simulink model "SPM_CellHarness"  (R2024b)
settings: Solver=ode15s  StartTime=0.0  StopTime=3600  FixedStep=1  MaxStep=1  RelTol=1e-4  AbsTol=1e-6
libraries: fl_lib x9, nesl_utility x5, BatteryCurrentManagement x1, batt_lib x1, BatteryEstimators x1
settings Model: Creator=annaf  LastModifiedBy=annaf

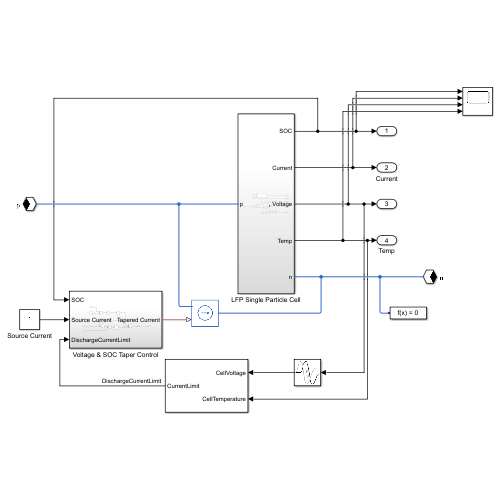
[thumbnail: Simulink's stored preview of the top-level diagram]
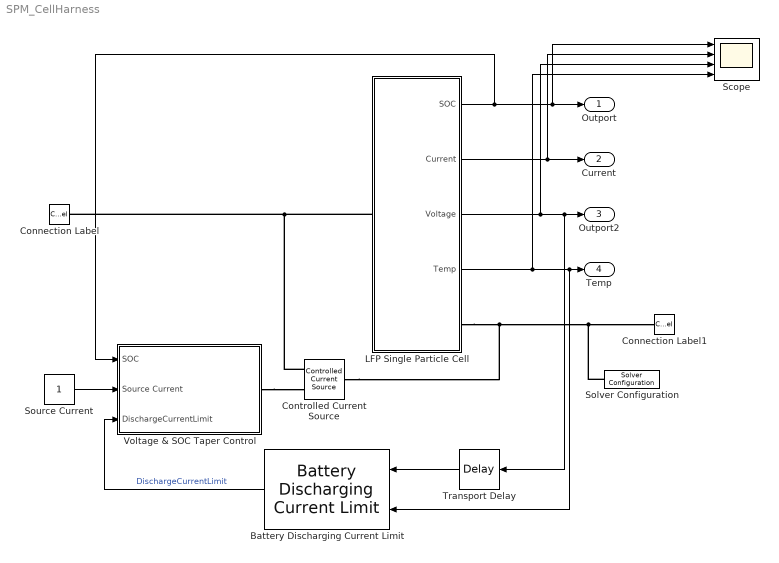
== system SPM_CellHarness ==
  Battery Discharging Current Limit : BatteryCurrentManagement/Battery Discharging Current Limit  CellUndervoltageLimit=3.2  R0=0.004  T_vec=[243.15, 258.15, 273.15, 288.15, 303.15, 318.15, 333.15]  CurrentLimitCoolestCell=[ 0, 0, 0, 0, 5, 5, 5]  CurrentLimitHottestCell=[5, 5, 5, 5, 0, 0, 0]
      settings: LibrarySourceBlock=|
      | batt_sl_lib/Current Management/Battery Discharging
      | Current Limit
  Connection Label : ConnectionLabel  Label=p
  Connection Label1 : ConnectionLabel  Label=n
  Controlled Current Source : fl_lib/Electrical/Electrical Sources/Controlled Current Source
  LFP Single Particle Cell : Subsystem
  Scope : Scope  NumInputPorts=4
  Solver Configuration : nesl_utility/Solver Configuration  PhysicalDomain=network_engine_domain  SubClassName=solver  LeftPortType=input  RightPortType=generic  Tones=[]  Harmonics=[]  SimulateNoise=off  Profile=off  UseLocalSampling=off  EnableSwitchedLinearOptims=on  FrequencyDomain=off  UseCCode=off  RelTol=0.001  AbsTol=0.001  MinStep=1e-09  ToWorkspace=off  RevertToSquareIcSolve=off  NumHomotopyIterations=100  PhasorMode=off  PhasorModeNumHarmonics=1  ConsistencySolver=NEWTON_XTOL_AFTER_FTOL  IndexReductionMethod=DerivativeReplacement  DoDC=off  ResidualTolerance=1e-09  ConsistencyTolSource=LOCAL  ConsistencyAbsTol=0.000001  ConsistencyRelTol=0.0001  ConsistencyTolFactor=0.001  UseLocalSolver=off  LocalSolverChoice=NE_BACKWARD_EULER_ADVANCER  ResolveIndetEquations=on  FunctionEvalNumThread=1  LocalSolverSampleTime=1  DoFixedCost=on  MaxNonlinIter=6  MaxModeIter=2  ComputeImpulses=off  ImpulseIterations=2  LinearAlgebra=Full  LinearAlgebraNumThread=0  EquationFormulation=NE_TIME_EF  DelaysMemoryBudget=1024  AutomaticFiltering=on  FilteringTimeConstant=0.001  PartitionStorageMethod=AS_NEEDED  PartitionMemoryBudget=1024  PartitionMethod=ROBUST  MultibodyUseLocalSolver=off  MultibodyLocalSolverChoice=ODE1  MultibodyLocalSolverSampleTime=0.001
  Source Current : Constant
  Transport Delay : TransportDelay  DelayTime=1e-6  TransDelayFeedthrough=on
  Voltage & SOC Taper Control : Subsystem
  Outport : Outport
  Current : Outport  Port=2
  Outport2 : Outport  Port=3
  Temp : Outport  Port=4
  wires:
  LFP Single Particle Cell/3(Voltage) -> Scope/3, Transport Delay/1, Outport2/1
  LFP Single Particle Cell/1(SOC) -> Scope/1, Outport/1, Voltage & SOC Taper Control/1(SOC)
  LFP Single Particle Cell/2(Current) -> Scope/2, Current/1
  LFP Single Particle Cell/4(Temp) -> Battery Discharging Current Limit/2, Temp/1, Scope/4
  Transport Delay/1 -> Battery Discharging Current Limit/1
  Battery Discharging Current Limit/1 -> Voltage & SOC Taper Control/3(DischargeCurrentLimit)  "DischargeCurrentLimit"
  Source Current/1 -> Voltage & SOC Taper Control/2(Source Current)
  connections:
  LFP Single Particle Cell/RConn1 -- Controlled Current Source/LConn1 -- Solver Configuration/RConn1 -- Connection Label1/LConn1
  LFP Single Particle Cell/LConn1 -- Controlled Current Source/RConn2 -- Connection Label/LConn1
  Voltage & SOC Taper Control/RConn1 -- Controlled Current Source/RConn1

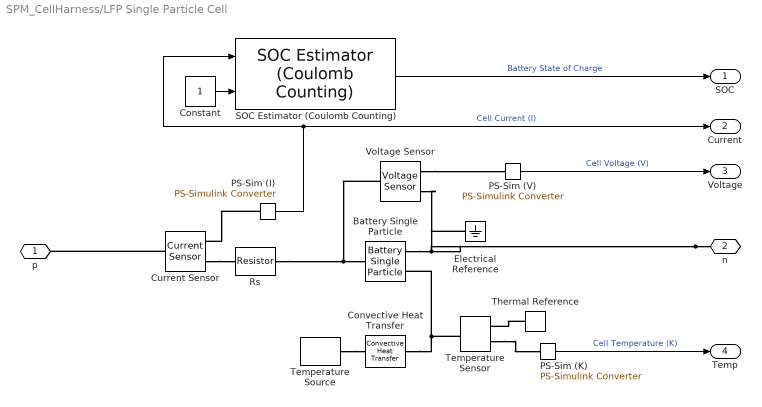
== system SPM_CellHarness/LFP Single Particle Cell ==
  Battery Single Particle : batt_lib/Cells/Electrochemical/Battery Single Particle  ExtrapolationMethod=simscape.enum.extrapolation.nearest  ThicknessAnode=3.4E-5 m  ElectrolyteLayerCountAnode=10  ThicknessSeparator=2.5E-5 m  ElectrolyteLayerCountSeparator=5  ThicknessCathode=8E-5 m  ElectrolyteLayerCountCathode=10  ElectrodePlateArea=1.5 m^2  ParticleRadiusAnode=5E-6 m  ShellCountAnode=40  ParticleRadiusCathode=5E-6 m  ShellCountCathode=40  ActiveMaterialVolumeFractionAnode=0.58  ActiveMaterialVolumeFractionCathode=0.374  OpenCircuitPotentialAnode=[0.200;0.180;0.160;0.140;0.120;0.110;0.102;0.098;0.094;0.092;0.091;0.090;0.089;0.089;0.088;0.088;0.088;0.088;0.088;0.088;0.088;0.087;0.087;0.087;0.086;0.086;0.085;0.085;0.084;0.084;0.083;0.083;0.082;0.082;0.081;0.081;0.080;0.079;0.078] V  OpenCircuitPotentialCathode=[3.200;3.280;3.340;3.380;3.410;3.420;3.425;3.430;3.432;3.433;3.434;3.435;3.435;3.436;3.436;3.437;3.437;3.438;3.438;3.439;3.439;3.440;3.440;3.441;3.441;3.442;3.442;3.443;3.443;3.444;3.444;3.445;3.446;3.447;3.448;3.449;3.460;3.480;3.500] V  NormalizedStoichiometryBreakpoints=linspace(0.025, 0.975, 39)  MaximumConcentrationAnode=30555 mol/m^3  MaximumStoichiometryAnode=0.811  MinimumStoichiometryAnode=0.0132  MaximumConcentrationCathode=22806 mol/m^3  MaximumStoichiometryCathode=0.74  MinimumStoichiometryCathode=0.035  ActiveMaterialDiffusionCoefficientAnode=3E-15 m^2/s  ActiveMaterialDiffusionCoefficientCathode=1E-15 m^2/s  ConductivityAnode=100 S/m  ConductivityCathode=0.5 S/m  CurrentCollectorResistance=1E-3 Ohm  ElectrolyteVolumeFractionAnode=0.3874  ElectrolyteVolumeFractionSeparator=0.45  ElectrolyteVolumeFractionCathode=0.5725  ElectrolyteConductivity=0.29 S/m  BruggemanExponentAnode=1.5  BruggemanExponentSeparator=1.5  BruggemanExponentCathode=1.5  TransferenceNumber=0.363  ElectrolyteDiffusionCoefficient=2E-10 m^2/s  ChargeTransferRateAnode=1E-9 m^(5/2)/(mol^(1/2)*s)  ChargeTransferRateCathode=1E-11 m^(5/2)/(mol^(1/2)*s)  BatteryThermalMass=77 J/K  ArrheniusReferenceTemperature=298.15 K  ActiveMaterialDiffusionActivationEnergyAnode=39000 J/mol  ActiveMaterialDiffusionActivationEnergyCathode=35000 J/mol  ElectrolyteDiffusionActivationEnergy=26600 J/mol  ConductivityActivationEnergyAnode=3000 J/mol  ConductivityActivationEnergyCathode=3000 J/mol  ElectrolyteConductivityActivationEnergy=11000 J/mol  ChargeTransferActivationEnergyAnode=13000 J/mol  ChargeTransferActivationEnergyCathode=20000 J/mol  batteryCurrent_specify=off  batteryCurrent_priority=None  batteryCurrent=0 A  batteryCurrent_nominal_specify=off  batteryCurrent_nominal_value=1  batteryCurrent_nominal_unit=A  batteryVoltage_specify=off  batteryVoltage_priority=None  batteryVoltage=0 V  batteryVoltage_nominal_specify=off  batteryVoltage_nominal_value=1  batteryVoltage_nominal_unit=V  averageElectrolyteConcentration_specify=off  averageElectrolyteConcentration_priority=High  averageElectrolyteConcentration=1200 mol/m^3  averageElectrolyteConcentration_nominal_specify=off  averageElectrolyteConcentration_nominal_value=1  averageElectrolyteConcentration_nominal_unit=mol/m^3  stateOfCharge_specify=off  stateOfCharge_priority=High  stateOfCharge=0.5  stateOfCharge_nominal_specify=off  stateOfCharge_nominal_value=1  stateOfCharge_nominal_unit=1  batteryTemperature_specify=off  batteryTemperature_priority=High  batteryTemperature=298.15 K  batteryTemperature_nominal_specify=off  batteryTemperature_nominal_value=1  batteryTemperature_nominal_unit=K
      settings: InternalSimscapePortConfiguration="{\"Bottom\":[],\"Left\":[{\"id\":\"p\",\"label\":\"+\",\"type\":\"foundation.electrical.electrical\"}],\"Right\":[{\"id\":\"n\",\"label\":\"-\",\"type\":\"foundation.electrical.electrical\"},{\"id\":\"H\",\"label\":\"H\",\"type\":\"foundation.thermal.thermal\"}],\"Top\":[]}"
  Constant : Constant
  Convective Heat Transfer : fl_lib/Thermal/Thermal Elements/Convective Heat Transfer  thermal_type=foundation.enum.constant_variable.constant  area=0.2 m^2  heat_tr_coeff=15 W/(K*m^2)  min_heat_tr_coeff=1e-3 W/(K*m^2)  T_specify=off  T_priority=None  T=0 K  T_nominal_specify=off  T_nominal_value=1  T_nominal_unit=K  Q_specify=on  Q_priority=None  Q=0 W  Q_nominal_specify=off  Q_nominal_value=1  Q_nominal_unit=W
  Current Sensor : fl_lib/Electrical/Electrical Sensors/Current Sensor
  Electrical Reference : fl_lib/Electrical/Electrical Elements/Electrical Reference
  PS-Sim (I) : nesl_utility/PS-Simulink Converter  PhysicalDomain=network_engine_domain  SubClassName=ps_output  LeftPortType=input  RightPortType=output  PseudoPeriodic=off  Frequencies=[]  VectorFormat=inherit  Unit=A  AffineConversion=off
  PS-Sim (K) : nesl_utility/PS-Simulink Converter  PhysicalDomain=network_engine_domain  SubClassName=ps_output  LeftPortType=input  RightPortType=output  PseudoPeriodic=off  Frequencies=[]  VectorFormat=inherit  Unit=K  AffineConversion=off
  PS-Sim (V) : nesl_utility/PS-Simulink Converter  PhysicalDomain=network_engine_domain  SubClassName=ps_output  LeftPortType=input  RightPortType=output  PseudoPeriodic=off  Frequencies=[]  VectorFormat=inherit  Unit=V  AffineConversion=off
  Rs : fl_lib/Electrical/Electrical Elements/Resistor  R=0.004 Ohm  i_specify=off  i_priority=None  i=0 A  i_nominal_specify=off  i_nominal_value=3  i_nominal_unit=A  v_specify=off  v_priority=None  v=0 V  v_nominal_specify=off  v_nominal_value=3.5  v_nominal_unit=V
  SOC Estimator (Coulomb Counting) : BatteryEstimators/SOC Estimator (Coulomb Counting)  CurrentInputPartition=on  AH=3  Ts=-1
      settings: LibrarySourceBlock=|
      | batt_sl_lib/Estimators/SOC Estimator
      | (Coulomb Counting)
  Temperature Sensor : fl_lib/Thermal/Thermal Sensors/Temperature Sensor  temperature_measure=foundation.enum.MeasurementReference.difference
  Temperature Source : fl_lib/Thermal/Thermal Sources/Temperature Source  temperature=298.15 K
  Thermal Reference : fl_lib/Thermal/Thermal Elements/Thermal Reference
  Voltage Sensor : fl_lib/Electrical/Electrical Sensors/Voltage Sensor
  p : PMIOPort  Side=Left
  n : PMIOPort  Port=2  Side=Right
  SOC : Outport
  Current : Outport  Port=2
  Voltage : Outport  Port=3
  Temp : Outport  Port=4
  wires:
  PS-Sim (K)/1 -> Temp/1  "Cell Temperature (K)"
  PS-Sim (I)/1 -> Current/1, SOC Estimator (Coulomb Counting)/1  "Cell Current (I)"
  PS-Sim (V)/1 -> Voltage/1  "Cell Voltage (V)"
  Constant/1 -> SOC Estimator (Coulomb Counting)/2
  SOC Estimator (Coulomb Counting)/1 -> SOC/1  "Battery State of Charge"
  connections:
  Rs/LConn1 -- Voltage Sensor/LConn1 -- Battery Single Particle/LConn1
  n/RConn1 -- Battery Single Particle/RConn1 -- Voltage Sensor/RConn2 -- Electrical Reference/LConn1
  Current Sensor/LConn1 -- p/RConn1
  Convective Heat Transfer/LConn1 -- Battery Single Particle/RConn2 -- Temperature Sensor/LConn1
  Voltage Sensor/RConn1 -- PS-Sim (V)/LConn1
  PS-Sim (I)/LConn1 -- Current Sensor/RConn1
  Current Sensor/RConn2 -- Rs/RConn1
  Thermal Reference/LConn1 -- Temperature Sensor/RConn1
  Temperature Source/LConn1 -- Convective Heat Transfer/RConn1
  Temperature Sensor/RConn2 -- PS-Sim (K)/LConn1

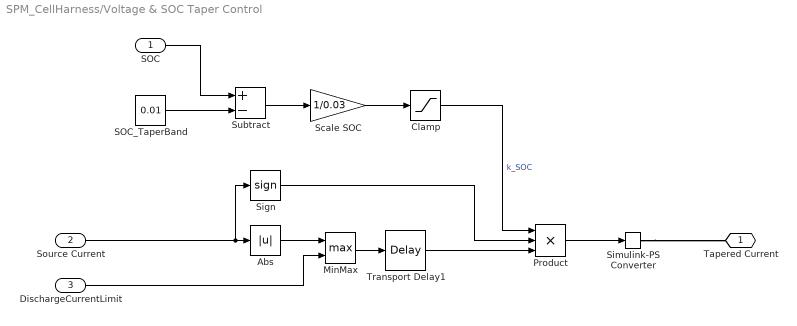
== system SPM_CellHarness/Voltage & SOC Taper Control ==
  SOC : Inport
  Source Current : Inport  Port=2
  DischargeCurrentLimit : Inport  Port=3
  Abs : Abs  SaturateOnIntegerOverflow=off
  Clamp : Saturate  UpperLimit=1  LowerLimit=0
  MinMax : MinMax  Function=max  Inputs=2
  Product : Product  Inputs=3
  SOC_TaperBand : Constant  Value=0.01
  Scale SOC : Gain  Gain=1/0.03
  Sign : Signum
  Simulink-PS Converter : nesl_utility/Simulink-PS Converter  PhysicalDomain=network_engine_domain  SubClassName=ps_input  LeftPortType=input  RightPortType=output  PseudoPeriodic=off  Frequencies=[]  NoiseDistribution=none  NoiseParameters=[]  Unit=A  AffineConversion=off  FilteringAndDerivatives=provide  SimscapeFilterOrder=1  InputFilterTimeConstant=0.001  UdotUserProvided=0
  Subtract : Sum  Inputs=+-
  Transport Delay1 : TransportDelay  DelayTime=1e-6  TransDelayFeedthrough=on
  Tapered Current : PMIOPort  Side=Right
  wires:
  Product/1 -> Simulink-PS Converter/1
  SOC_TaperBand/1 -> Subtract/2
  Source Current/1 -> Sign/1, Abs/1
  Transport Delay1/1 -> Product/3
  Subtract/1 -> Scale SOC/1
  Scale SOC/1 -> Clamp/1
  MinMax/1 -> Transport Delay1/1
  Abs/1 -> MinMax/1
  Sign/1 -> Product/2
  Clamp/1 -> Product/1  "k_SOC"
  SOC/1 -> Subtract/1
  DischargeCurrentLimit/1 -> MinMax/2
  connections:
  Simulink-PS Converter/RConn1 -- Tapered Current/RConn1
